simulink model "sampleModel1465"  (R2023a)
settings: Solver=VariableStepAuto  StartTime=0.0  StopTime=10.0  RelTol=1e-3
libraries: hdlsllib x5
settings Model: Creator=user1  LastModifiedBy=user1

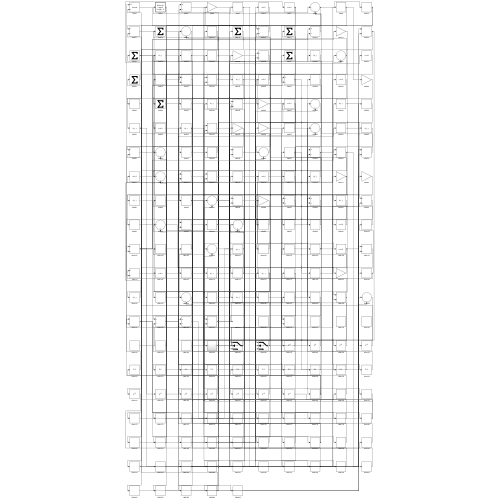
[thumbnail: Simulink's stored preview of the top-level diagram]
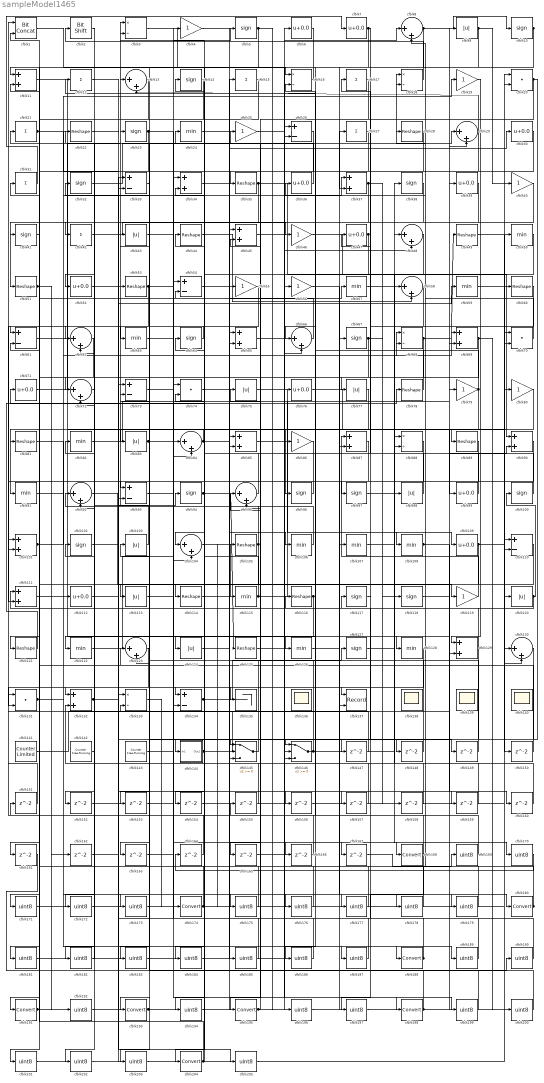
== system sampleModel1465 ==
  cfblk1 : hdlsllib/Logic and Bit Operations/Bit Concat  numInputs=2
  cfblk{5,10,14,23,32,38,41,64,67,94,96..97,100,102,117..118,127} (17 alike) : Signum
  cfblk{11,34,37,45,65,69,85,87,90,101,111,129,132} (13 alike) : Sum
  cfblk{9,43,75,77,83,98,103,113,120,124} (10 alike) : Abs  SaturateOnIntegerOverflow=off
  cfblk{8,13,29,48,58,62,66,72,84,92,95,104,123,130} (14 alike) : Sum  Inputs=|++
  cfblk{22,28,35,44,49,51,53,60,78,81,89,105,114,116,121,125} (16 alike) : Reshape
  cfblk{24,50,57,59,63,82,91,106..108,115,122,126,128} (14 alike) : MinMax
  cfblk{6..7,30,36,39,47,52,71,76,99,109,112} (12 alike) : Bias  Bias=0.0  SaturateOnIntegerOverflow=off
  cfblk{26,33,54,61,73,93,110,134} (8 alike) : Sum  Inputs=+-
  cfblk{4,19,25,40,46,55..56,79..80,86,119} (11 alike) : Gain
  cfblk{12,15,17,21,27,31,42} (7 alike) : Sum  Inputs=+
  cfblk{20,70,74,131} (4 alike) : DotProduct  OutDataTypeStr=Inherit: Inherit via internal rule
  cfblk{3,16,18,68,88,133} (6 alike) : Product  Inputs=*/  RndMeth=Zero  SaturateOnIntegerOverflow=on
  cfblk135 : Terminator
  cfblk{136,138..140} (4 alike) : Scope
      settings: Floating=on
  cfblk137 : Record  FileSettingsInternal="{\"entries\":[{\"content\":{\"excelSettings\":{\"content\":{},\"type\":\"Streamout.ExcelSettings\"}},\"type\":\"Streamout.FileSettingStorage\",\"uuid\":\"\"}],\"packageUris\":[\"http:\\/\\/schema.mathworks.com\\/mf0\\/streamout_blocks\\/R2020a\"],\"version\":\"1.0\"}"  Layout=[1 1]  SignalsInternal="{\"entries\":[{\"content\":{\"signals\":[{\"content\":{\"blockPath\":[],\"dimensions\":[1],\"domain\":\"\",\"lineColor\":\"#a2142f\",\"plots\":[1],\"port\":1,\"signalID\":873,\"signalName\":\"XY Graph:1\"},\"type\":\"RecordBlkView.Signal\",\"uuid\":\"\"},{\"content\":{\"blockPath\":[],\"dimensions\":[1],\"domain\":\"\",\"lineColor\":\"#139fff\",\"plots\":[1],\"port\":2,\"signalID\":876,\"signalName\":\"XY Graph:2\"},\"type\":\"RecordBlkView.Signal\",\"uuid\":\"\"}]},\"type\":\"RecordBlkView.InputSignals\",\"uuid\":\"\"}],\"packageUris\":[\"http:\\/\\/schema.mathworks.com\\/mf0\\/streamout_blocks\\/R2020a\"],\"version\":\"1.0\"}"  VisualizationBindings="{\"xyplotplugin\":{\"info\":[{\"series\":[{\"bindingParametersList\":[{\"parameter\":\"X-Axis\",\"signalID\":873,\"signalName\":\"XY Graph:1\"},{\"parameter\":\"Y-Axis\",\"signalID\":876,\"signalName\":\"XY Graph:2\"}],\"seriesID\":38834}],\"subplotID\":1}]}}"  CompatibilityTag=XY  st=-1
  cfblk141 : hdlsllib/Sources/Counter Limited  uplimit=7  tsamp=-1
  cfblk142 : hdlsllib/Sources/Counter Free-Running  NumBits=16  tsamp=-1
  cfblk143 : hdlsllib/Sources/Counter Free-Running  NumBits=16  tsamp=-1
  cfblk144 : Subsystem
      settings: LibrarySourceBlock=|
      | hdlsllib/Ports &
      | Subsystems/Subsystem
  cfblk145 : Switch  SaturateOnIntegerOverflow=off  InputSameDT=off
  cfblk146 : Switch  SaturateOnIntegerOverflow=off  InputSameDT=off
  cfblk{147..167} (21 alike) : Delay  SampleTime=1
  cfblk{168,174,180,188,191,193,195,198,204} (9 alike) : DataTypeConversion  SaturateOnIntegerOverflow=off  RndMeth=Floor
  cfblk{169..173,175..179,181..187,189..190,192,194,196..197,199..203,205} (29 alike) : DataTypeConversion  OutDataTypeStr=uint8  SaturateOnIntegerOverflow=off  RndMeth=Floor
  cfblk2 : hdlsllib/Logic and Bit Operations/Bit Shift  mode=Shift Left Logical  N=0
  wires:
  cfblk119/1 -> cfblk87/1
  cfblk36/1 -> cfblk21/1
  cfblk120/1 -> cfblk111/1, cfblk100/1
  cfblk18/1 -> cfblk2/1
  cfblk121/1 -> cfblk78/1
  cfblk105/1 -> cfblk3/1, cfblk145/3
  cfblk80/1 -> cfblk193/1
  cfblk83/1 -> cfblk148/1, cfblk199/1
  cfblk60/1 -> cfblk97/1
  cfblk134/1 -> cfblk127/1, cfblk68/2
  cfblk59/1 -> cfblk90/1
  cfblk20/1 -> cfblk144/1(In1), cfblk165/1
  cfblk79/1 -> cfblk89/1, cfblk17/1, cfblk96/1
  cfblk92/1 -> cfblk119/1
  cfblk116/1 -> cfblk122/1, cfblk194/1
  cfblk127/1 -> cfblk48/1
  cfblk8/1 -> cfblk10/1, cfblk203/1
  cfblk97/1 -> cfblk58/1
  cfblk145/1 -> cfblk103/1
  cfblk64/1 -> cfblk63/1
  cfblk117/1 -> cfblk137/1
  cfblk73/1 -> cfblk188/1
  cfblk35/1 -> cfblk98/1, cfblk145/2
  cfblk11/1 -> cfblk128/1
  cfblk21/1 -> cfblk137/2, cfblk33/2
  cfblk39/1 -> cfblk51/1
  cfblk96/1 -> cfblk93/1
  cfblk77/1 -> cfblk91/1
  cfblk75/1 -> cfblk109/1
  cfblk31/1 -> cfblk7/1
  cfblk5/1 -> cfblk171/1, cfblk196/1
  cfblk109/1 -> cfblk70/1, cfblk145/1
  cfblk103/1 -> cfblk82/1
  cfblk94/1 -> cfblk125/1, cfblk44/1
  cfblk28/1 -> cfblk126/1
  cfblk61/1 -> cfblk99/1
  cfblk132/1 -> cfblk59/1, cfblk205/1
  cfblk17/1 -> cfblk146/1
  cfblk14/1 -> cfblk41/1
  cfblk71/1 -> cfblk13/1
  cfblk124/1 -> cfblk57/1
  cfblk44/1 -> cfblk58/2
  cfblk106/1 -> cfblk92/1
  cfblk130/1 -> cfblk195/1
  cfblk40/1 -> cfblk114/1
  cfblk125/1 -> cfblk48/2
  cfblk141/1 -> cfblk76/1
  cfblk104/1 -> cfblk115/1
  cfblk68/1 -> cfblk49/1, cfblk81/1
  cfblk37/1 -> cfblk52/1, cfblk158/1
  cfblk10/1 -> cfblk104/1, cfblk37/2
  cfblk19/1 -> cfblk129/1
  cfblk50/1 -> cfblk204/1
  cfblk46/1 -> cfblk60/1
  cfblk62/1 -> cfblk72/1
  cfblk91/1 -> cfblk37/1
  cfblk48/1 -> cfblk66/1
  cfblk133/1 -> cfblk174/1
  cfblk53/1 -> cfblk111/2, cfblk157/1
  cfblk115/1 -> cfblk9/1, cfblk64/1
  cfblk76/1 -> cfblk120/1
  cfblk98/1 -> cfblk14/1
  cfblk114/1 -> cfblk29/1
  cfblk122/1 -> cfblk5/1
  cfblk131/1 -> cfblk173/1, cfblk189/1
  cfblk3/1 -> cfblk146/2
  cfblk2/1 -> cfblk62/1
  cfblk118/1 -> cfblk90/2
  cfblk78/1 -> cfblk12/1
  cfblk42/1 -> cfblk46/1
  cfblk24/1 -> cfblk88/2
  cfblk89/1 -> cfblk95/2
  cfblk56/1 -> cfblk180/1
  cfblk12/1 -> cfblk124/1
  cfblk7/1 -> cfblk77/1, cfblk202/1
  cfblk16/1 -> cfblk11/1
  cfblk25/1 -> cfblk168/1
  cfblk63/1 -> cfblk4/1
  cfblk90/1 -> cfblk134/1
  cfblk113/1 -> cfblk84/2
  cfblk70/1 -> cfblk36/1
  cfblk30/1 -> cfblk123/2
  cfblk84/1 -> cfblk15/1, cfblk83/1, cfblk106/1
  cfblk95/1 -> cfblk71/1
  cfblk45/1 -> cfblk198/1
  cfblk65/1 -> cfblk8/1
  cfblk33/1 -> cfblk113/1
  cfblk99/1 -> cfblk47/1
  cfblk29/1 -> cfblk61/1, cfblk13/2
  cfblk108/1 -> cfblk68/1, cfblk160/1
  cfblk47/1 -> cfblk135/1, cfblk154/1
  cfblk143/1 -> cfblk134/2
  cfblk23/1 -> cfblk92/2, cfblk85/2
  cfblk81/1 -> cfblk112/1
  cfblk67/1 -> cfblk93/2, cfblk118/1
  cfblk146/1 -> cfblk32/1, cfblk38/1
  cfblk85/1 -> cfblk108/1
  cfblk51/1 -> cfblk161/1, cfblk162/1
  cfblk82/1 -> cfblk29/2
  cfblk32/1 -> cfblk18/1
  cfblk55/1 -> cfblk191/1
  cfblk15/1 -> cfblk42/1
  cfblk27/1 -> cfblk35/1
  cfblk41/1 -> cfblk121/1
  cfblk1/1 -> cfblk16/1
  cfblk101/1 -> cfblk69/1, cfblk19/1, cfblk18/2, cfblk192/1
  cfblk129/1 -> cfblk116/1, cfblk163/1
  cfblk88/1 -> cfblk101/2
  cfblk142/1 -> cfblk72/2
  cfblk66/1 -> cfblk31/1
  cfblk123/1 -> cfblk131/2
  cfblk144/1(Out1) -> cfblk27/1, cfblk79/1
  cfblk69/1 -> cfblk87/2, cfblk200/1
  cfblk128/1 -> cfblk132/1
  cfblk74/1 -> cfblk30/1
  cfblk9/1 -> cfblk40/1, cfblk186/1
  cfblk112/1 -> cfblk94/1
  cfblk100/1 -> cfblk3/2
  cfblk57/1 -> cfblk129/2
  cfblk58/1 -> cfblk147/1
  cfblk147/1 -> cfblk131/1
  cfblk148/1 -> cfblk65/1
  cfblk102/1 -> cfblk149/1
  cfblk149/1 -> cfblk74/2
  cfblk49/1 -> cfblk150/1
  cfblk150/1 -> cfblk11/2
  cfblk151/1 -> cfblk1/1
  cfblk72/1 -> cfblk152/1
  cfblk152/1 -> cfblk84/1
  cfblk38/1 -> cfblk153/1
  cfblk154/1 -> cfblk66/2
  cfblk155/1 -> cfblk123/1
  cfblk22/1 -> cfblk156/1
  cfblk156/1 -> cfblk70/2
  cfblk157/1 -> cfblk132/2
  cfblk158/1 -> cfblk88/1
  cfblk52/1 -> cfblk159/1
  cfblk159/1 -> cfblk85/1
  cfblk160/1 -> cfblk8/2
  cfblk162/1 -> cfblk33/1
  cfblk163/1 -> cfblk104/2
  cfblk164/1 -> cfblk1/2
  cfblk4/1 -> cfblk166/1
  cfblk166/1 -> cfblk101/1
  cfblk43/1 -> cfblk167/1
  cfblk168/1 -> cfblk16/2, cfblk62/2, cfblk43/1, cfblk197/1
  cfblk167/1 -> cfblk169/1
  cfblk169/1 -> cfblk25/1
  cfblk107/1 -> cfblk170/1
  cfblk170/1 -> cfblk164/1
  cfblk171/1 -> cfblk107/1
  cfblk6/1 -> cfblk172/1
  cfblk172/1 -> cfblk20/1
  cfblk173/1 -> cfblk6/1
  cfblk174/1 -> cfblk151/1, cfblk105/1
  cfblk153/1 -> cfblk175/1
  cfblk175/1 -> cfblk133/1
  cfblk111/1 -> cfblk176/1
  cfblk176/1 -> cfblk133/2
  cfblk34/1 -> cfblk177/1
  cfblk177/1 -> cfblk22/1
  cfblk126/1 -> cfblk178/1
  cfblk178/1 -> cfblk34/1
  cfblk93/1 -> cfblk179/1
  cfblk179/1 -> cfblk34/2
  cfblk180/1 -> cfblk155/1, cfblk28/1
  cfblk13/1 -> cfblk181/1
  cfblk181/1 -> cfblk56/1
  cfblk26/1 -> cfblk182/1
  cfblk182/1 -> cfblk102/1
  cfblk86/1 -> cfblk183/1
  cfblk183/1 -> cfblk26/1
  cfblk87/1 -> cfblk184/1
  cfblk184/1 -> cfblk26/2
  cfblk54/1 -> cfblk185/1
  cfblk185/1 -> cfblk74/1
  cfblk186/1 -> cfblk54/1
  cfblk165/1 -> cfblk187/1
  cfblk187/1 -> cfblk54/2
  cfblk188/1 -> cfblk117/1, cfblk75/1
  cfblk189/1 -> cfblk73/1
  cfblk161/1 -> cfblk190/1
  cfblk190/1 -> cfblk73/2
  cfblk191/1 -> cfblk20/2, cfblk65/2
  cfblk192/1 -> cfblk55/1
  cfblk193/1 -> cfblk69/2, cfblk146/3, cfblk67/1
  cfblk194/1 -> cfblk80/1
  cfblk195/1 -> cfblk86/1, cfblk95/1
  cfblk196/1 -> cfblk130/1
  cfblk197/1 -> cfblk130/2
  cfblk198/1 -> cfblk39/1, cfblk23/1
  cfblk199/1 -> cfblk45/1
  cfblk200/1 -> cfblk45/2
  cfblk110/1 -> cfblk201/1
  cfblk201/1 -> cfblk53/1
  cfblk202/1 -> cfblk110/1
  cfblk203/1 -> cfblk110/2
  cfblk204/1 -> cfblk61/2, cfblk24/1
  cfblk205/1 -> cfblk50/1

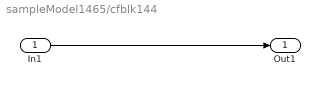
== system sampleModel1465/cfblk144 ==
  In1 : Inport
  Out1 : Outport
  wires:
  In1/1 -> Out1/1
